simulink model "Scaling"  (R2018a)
settings: Solver=VariableStepAuto  StartTime=0.0  StopTime=60  RelTol=1e-3
libraries: simulink x1
settings Model: Creator=hanistom  LastModifiedBy=efrem

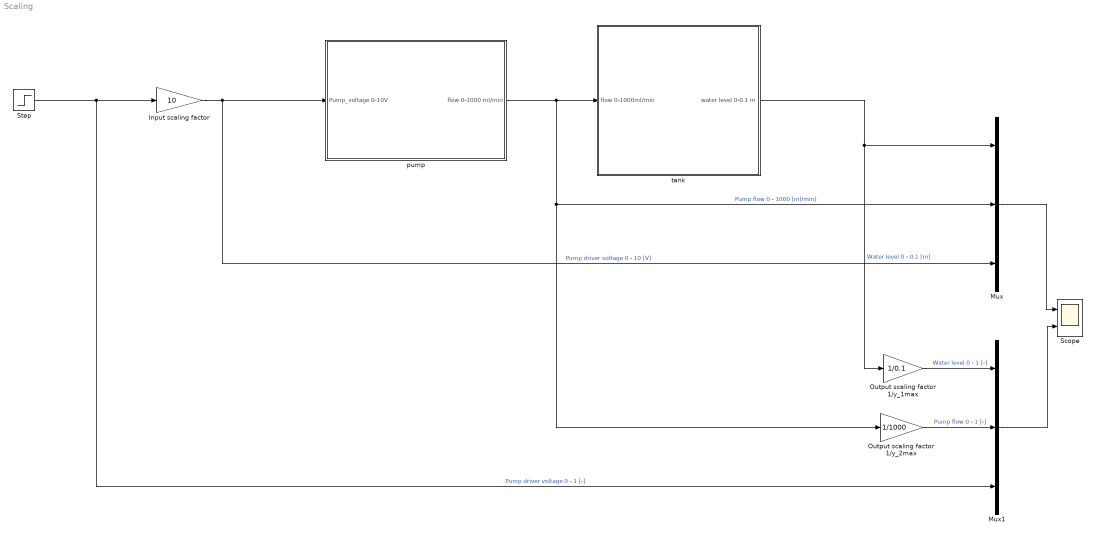
== system Scaling ==
  Input scaling factor : Gain  Gain=10
  Mux : Mux  Inputs=3
  Mux1 : Mux  Inputs=3
  Output scaling factor 1/y_1max : Gain  Gain=1/0.1
  Output scaling factor 1/y_2max : Gain  Gain=1/1000
  Scope : Scope  NumInputPorts=2
  Step : Step  After=0.5  SampleTime=0
  pump : Subsystem
      mask Display: image('.\Figure\pump.gif')
  tank : Subsystem
      mask Display: image('.\Figure\tank-schematic.jpg')
  wires:
  Mux/1 -> Scope/1
  pump/1(flow 0-1000 ml/min) -> tank/1(flow 0-1000ml/min), Output scaling factor 1/y_2max/1, Mux/2  "Pump flow 0 - 1000 [ml/min]"
  tank/1(water level 0-0.1 m) -> Output scaling factor 1/y_1max/1, Mux/1  "Water level 0 - 0.1 [m]"
  Mux1/1 -> Scope/2
  Output scaling factor 1/y_1max/1 -> Mux1/1  "Water level 0 - 1 [-]"
  Output scaling factor 1/y_2max/1 -> Mux1/2  "Pump flow 0 - 1 [-]"
  Step/1 -> Input scaling factor/1, Mux1/3  "Pump driver voltage 0 - 1 [-]"
  Input scaling factor/1 -> pump/1(Pump_voltage 0-10V), Mux/3  "Pump driver voltage 0 - 10 [V]"

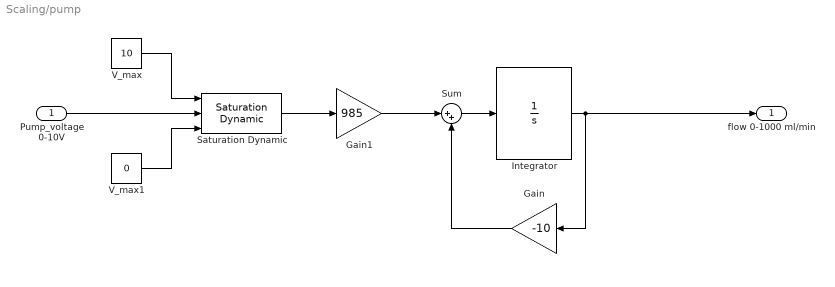
== system Scaling/pump ==
  Pump_voltage 0-10V : Inport
  Gain : Gain  Gain=-10
  Gain1 : Gain  Gain=985
  Integrator : Integrator  LimitOutput=on  UpperSaturationLimit=1000  LowerSaturationLimit=0
  Saturation Dynamic : simulink/Discontinuities/Saturation Dynamic  OutMin=[]  OutMax=[]  OutDataTypeStr=Inherit: Same as second input  OutDataType=fixdt(1, 16)  OutScaling=2^-10  DoSatur=off
  Sum : Sum  Inputs=|++
  V_max : Constant  Value=10
  V_max1 : Constant  Value=0
  flow 0-1000 ml/min : Outport
  wires:
  Gain/1 -> Sum/2
  Gain1/1 -> Sum/1
  V_max/1 -> Saturation Dynamic/1
  Integrator/1 -> flow 0-1000 ml/min/1, Gain/1
  V_max1/1 -> Saturation Dynamic/3
  Sum/1 -> Integrator/1
  Saturation Dynamic/1 -> Gain1/1
  Pump_voltage 0-10V/1 -> Saturation Dynamic/2

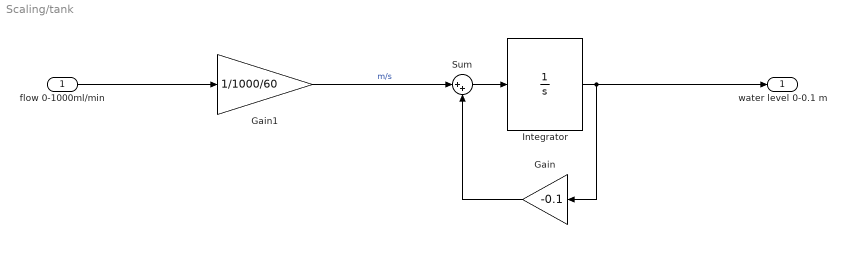
== system Scaling/tank ==
  flow 0-1000ml/min : Inport
  Gain : Gain  Gain=-0.1
  Gain1 : Gain  Gain=1/1000/60
  Integrator : Integrator  LimitOutput=on  UpperSaturationLimit=0.1  LowerSaturationLimit=0
  Sum : Sum  Inputs=|++
  water level 0-0.1 m : Outport
  wires:
  flow 0-1000ml/min/1 -> Gain1/1
  Sum/1 -> Integrator/1
  Integrator/1 -> Gain/1, water level 0-0.1 m/1
  Gain1/1 -> Sum/1  "m/s"
  Gain/1 -> Sum/2
